simulink model "Problem_2"  (R2020b)
settings: Solver=VariableStepAuto  StartTime=0.0  StopTime=10.0  RelTol=1e-3
model workspace (MAT data in the model file):
  b = 50
  k = 100
  k1 = 25
  k2 = 50
settings Model: Creator=Saqlain  LastModifiedBy=mluser

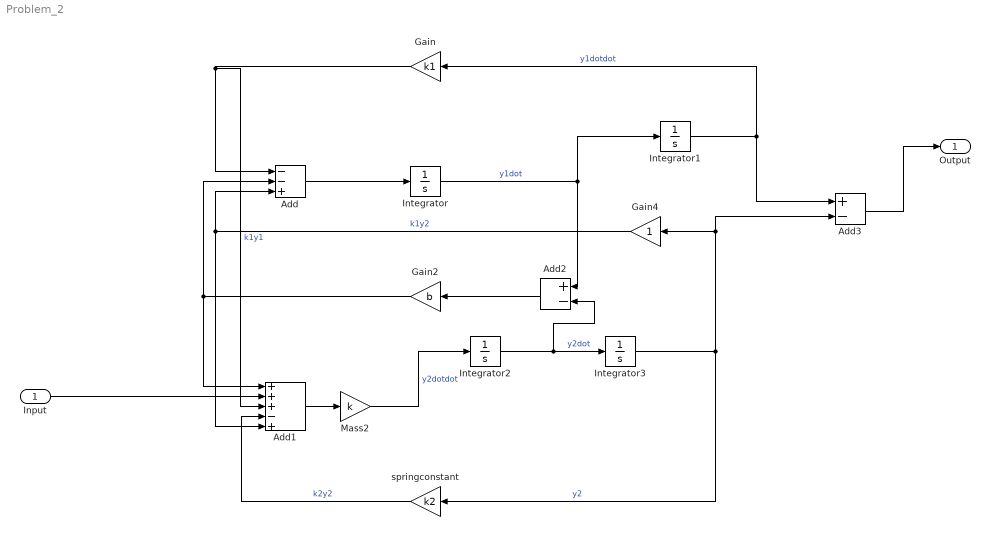
== system Problem_2 ==
  Input : Inport
  Add : Sum  Inputs=--+
  Add1 : Sum  Inputs=+++-+
  Add2 : Sum  Inputs=+-
  Add3 : Sum  Inputs=+-
  Gain : Gain  Gain=k1
  Gain2 : Gain  Gain=b
  Gain4 : Gain
  Integrator{,1..3} (4 alike) : Integrator
  Mass2 : Gain  Gain=k
  springconstant : Gain  Gain=k2
  Output : Outport
  wires:
  springconstant/1 -> Add1/4  "k2y2"
  Add2/1 -> Gain2/1
  Input/1 -> Add1/2
  Gain/1 -> Add1/3, Add/1  "k1y1"
  Mass2/1 -> Integrator2/1  "y2dotdot"
  Gain2/1 -> Add1/1, Add/2
  Integrator1/1 -> Gain/1, Add3/1  "y1dotdot"
  Add3/1 -> Output/1
  Integrator3/1 -> springconstant/1, Add3/2, Gain4/1  "y2"
  Add/1 -> Integrator/1
  Add1/1 -> Mass2/1
  Gain4/1 -> Add1/5, Add/3  "k1y2"
  Integrator/1 -> Add2/1, Integrator1/1  "y1dot"
  Integrator2/1 -> Add2/2, Integrator3/1  "y2dot"
